simulink model "DC_Model_Collect"  (R2018a)
settings: Solver=VariableStepAuto  StartTime=0.0  StopTime=10.0  RelTol=1e-3
values from neighbouring files (symbols this model uses):
  A = [0 1 ; 0 -1]    [Ch8_18.m]    (also in Ch8_24.m = [-2 1; 0 -2]; Ch8_26.m = [1 0 ; 1 1]; DCT_3_3.m = find(abs(Zd)<0.05); DC_Model.m = [0 1 0; 0 -(B/J) Kt/J; 0 -(Ke/L) -(R/L)])
  a = 1:0.1:1.5    [Ch7_19.m]    (also in Ch7_25.m = (1-sin(th))/(1+sin(th)); DC_Model.m = 1)
  B = [1 ; 1]    [Ch8_18.m]    (also in Ch8_24.m = [1; 1]; Ch8_26.m = B0+expm(-A)*B1; DC_Model.m = 6.2e-05; NpointFFT.m = zeros(1,z-length(x)))
  B1 = [0; B]    [Ch8_24.m]    (also in Ch8_26.m = [0 ; 1]; DC_Model.m = [0; 0; 1/L])
  C = [2 1]    [Ch8_18.m]    (also in Ch8_24.m = [1 1]; Ch8_26.m = [1 1]; DC_Model.m = [1 0 0])
  J = 31*10^(-6)    (= 3.1e-05)    [DC_Model.m]
  Ka = 1/(3*Kp)    (= 0.0265223848928)    [DC_Model.m]
  Kas = 1/Kps    (= 110.951304705)    [DC_Model.m]
  Ke = 0.54    [DC_Model.m]
  Ki = R*1571    (= 3142)    [DC_Model.m]
  Kis = J*157^2/(5*Kt)    (= 0.283007037037)    [DC_Model.m]
  Kp = L*1571    (= 12.568)    [DC_Model.m]
  Kps = J*157/Kt    (= 0.00901296296296)    [DC_Model.m]
  Kps_1 = (1-a)*Kps    (= 0)    [DC_Model.m]
  Kt = 0.54    [DC_Model.m]
  L = 0.008    [DC_Model.m]
  posKa = 0    [DC_Model.m]
  posKd = 1    [DC_Model.m]
  posKi = 0    [DC_Model.m]
  posKp = 30    [DC_Model.m]
  R = 2    [Ch8_18.m]    (also in Ch8_26.m = 1; DC_Model.m)
undefined symbols (not defined in the file or in its folder): K
settings Model: Creator=admin  LastModifiedBy=admin

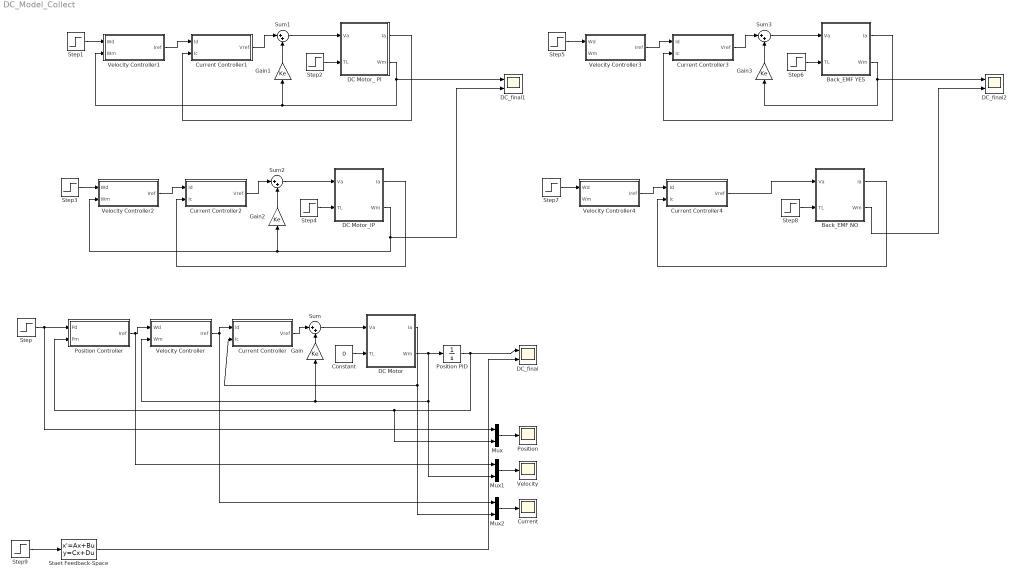
== system DC_Model_Collect ==
  Back_EMF NO : Subsystem
  Back_EMF YES : Subsystem
  Constant : Constant  Value=0
  Current : Scope
  Current Controller : Subsystem
  Current Controller1 : Subsystem
  Current Controller2 : Subsystem
  Current Controller3 : Subsystem
  Current Controller4 : Subsystem
  DC Motor : Subsystem
  DC Motor_ PI : Subsystem
  DC Motor_IP : Subsystem
  DC_final : Scope  NumInputPorts=2
  DC_final1 : Scope  NumInputPorts=2
  DC_final2 : Scope  NumInputPorts=2
  Gain{,1..3} (4 alike) : Gain  Gain=Ke
  Mux : Mux  Inputs=2
  Mux1 : Mux  Inputs=2
  Mux2 : Mux  Inputs=2
  Position : Scope
  Position Controller : Subsystem
  Position PID : Integrator
  Staet Feedback-Space : StateSpace  A=A-B1*K  B=B1  C=C  D=0  InitialCondition=0
  Step{,1,3,5,7,9} (6 alike) : Step  After=31.4  SampleTime=0
  Step{2,4,6,8} (4 alike) : Step  Time=2  After=0.1  SampleTime=0
  Sum{,1..3} (4 alike) : Sum  Inputs=|++
  Velocity : Scope
  Velocity Controller : Subsystem
  Velocity Controller1 : Subsystem
  Velocity Controller2 : Subsystem
  Velocity Controller3 : Subsystem
  Velocity Controller4 : Subsystem
  wires:
  Velocity Controller/1(Iref) -> Mux2/1, Current Controller/1(Id)
  DC Motor/2(Wm) -> Gain/1, Velocity Controller/2(Wm), Mux1/2, Position PID/1
  Position Controller/1(Iref) -> Mux1/1, Velocity Controller/1(Wd)
  Step/1 -> Mux/1, Position Controller/1(Pd)
  Position PID/1 -> DC_final/1, Position Controller/2(Pm), Mux/2
  DC Motor/1(Ia) -> Current Controller/2(Ic), Mux2/2
  Mux/1 -> Position/1
  Mux1/1 -> Velocity/1
  Mux2/1 -> Current/1
  Sum/1 -> DC Motor/1(Va)
  Gain/1 -> Sum/2
  Current Controller/1(Vref) -> Sum/1
  Sum1/1 -> DC Motor_ PI/1(Va)
  Step1/1 -> Velocity Controller1/1(Wd)
  Velocity Controller1/1(Iref) -> Current Controller1/1(Id)
  Current Controller1/1(Vref) -> Sum1/1
  Gain1/1 -> Sum1/2
  Step2/1 -> DC Motor_ PI/2(TL)
  DC Motor_ PI/1(Ia) -> Current Controller1/2(Ic)
  DC Motor_ PI/2(Wm) -> DC_final1/1, Gain1/1, Velocity Controller1/2(Wm)
  DC Motor_IP/2(Wm) -> DC_final1/2, Velocity Controller2/2(Wm), Gain2/1
  DC Motor_IP/1(Ia) -> Current Controller2/2(Ic)
  Step4/1 -> DC Motor_IP/2(TL)
  Gain2/1 -> Sum2/2
  Current Controller2/1(Vref) -> Sum2/1
  Velocity Controller2/1(Iref) -> Current Controller2/1(Id)
  Step3/1 -> Velocity Controller2/1(Wd)
  Sum2/1 -> DC Motor_IP/1(Va)
  Step7/1 -> Velocity Controller4/1(Wd)
  Velocity Controller4/1(Iref) -> Current Controller4/1(Id)
  Step8/1 -> Back_EMF NO/2(TL)
  Back_EMF NO/1(Ia) -> Current Controller4/2(Ic)
  Back_EMF NO/2(Wm) -> DC_final2/2
  Back_EMF YES/2(Wm) -> Gain3/1, DC_final2/1
  Back_EMF YES/1(Ia) -> Current Controller3/2(Ic)
  Step6/1 -> Back_EMF YES/2(TL)
  Gain3/1 -> Sum3/2
  Current Controller3/1(Vref) -> Sum3/1
  Velocity Controller3/1(Iref) -> Current Controller3/1(Id)
  Step5/1 -> Velocity Controller3/1(Wd)
  Sum3/1 -> Back_EMF YES/1(Va)
  Current Controller4/1(Vref) -> Back_EMF NO/1(Va)
  Step9/1 -> Staet Feedback-Space/1
  Constant/1 -> DC Motor/2(TL)
  Staet Feedback-Space/1 -> DC_final/2

== system DC_Model_Collect/Back_EMF NO ==
  Va : Inport
  TL : Inport  Port=2
  Gain : Gain  Gain=Kt
  Gain1 : Gain  Gain=Ke
  Sum : Sum  Inputs=|+-
  Sum1 : Sum  Inputs=-+|
  Transfer Fcn : TransferFcn  Denominator=[L R]
  Transfer Fcn1 : TransferFcn  Denominator=[J B]
  Ia : Outport
  Wm : Outport  Port=2
  wires:
  Va/1 -> Sum/1
  Transfer Fcn1/1 -> Wm/1, Gain1/1
  Sum/1 -> Transfer Fcn/1
  Gain/1 -> Sum1/2
  Sum1/1 -> Transfer Fcn1/1
  Gain1/1 -> Sum/2
  Transfer Fcn/1 -> Gain/1, Ia/1
  TL/1 -> Sum1/1

== system DC_Model_Collect/Back_EMF YES ==
  Va : Inport
  TL : Inport  Port=2
  Gain : Gain  Gain=Kt
  Gain1 : Gain  Gain=Ke
  Sum : Sum  Inputs=|+-
  Sum1 : Sum  Inputs=-+|
  Transfer Fcn : TransferFcn  Denominator=[L R]
  Transfer Fcn1 : TransferFcn  Denominator=[J B]
  Ia : Outport
  Wm : Outport  Port=2
  wires:
  TL/1 -> Sum1/1
  Transfer Fcn/1 -> Ia/1, Gain/1
  Gain1/1 -> Sum/2
  Sum1/1 -> Transfer Fcn1/1
  Gain/1 -> Sum1/2
  Sum/1 -> Transfer Fcn/1
  Transfer Fcn1/1 -> Gain1/1, Wm/1
  Va/1 -> Sum/1

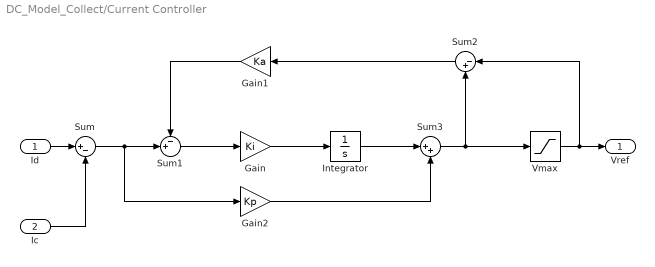
== system DC_Model_Collect/Current Controller ==
  Id : Inport
  Ic : Inport  Port=2
  Gain : Gain  Gain=Ki
  Gain1 : Gain  Gain=Ka
  Gain2 : Gain  Gain=Kp
  Integrator : Integrator
  Sum : Sum  Inputs=|+-
  Sum1 : Sum  Inputs=-+|
  Sum2 : Sum  Inputs=|-+
  Sum3 : Sum  Inputs=|++
  Vmax : Saturate  UpperLimit=200
  Vref : Outport
  wires:
  Id/1 -> Sum/1
  Sum1/1 -> Gain/1
  Ic/1 -> Sum/2
  Sum/1 -> Gain2/1, Sum1/2
  Gain1/1 -> Sum1/1
  Sum2/1 -> Gain1/1
  Vmax/1 -> Sum2/1, Vref/1
  Sum3/1 -> Sum2/2, Vmax/1
  Integrator/1 -> Sum3/1
  Gain/1 -> Integrator/1
  Gain2/1 -> Sum3/2

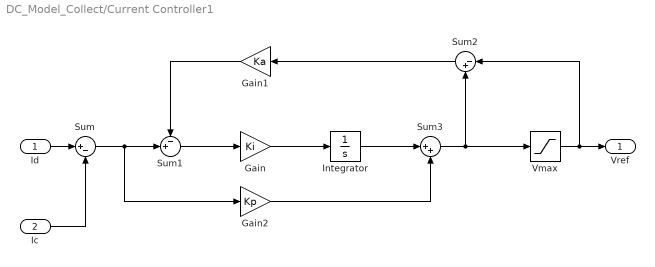
== system DC_Model_Collect/Current Controller1 ==
  Id : Inport
  Ic : Inport  Port=2
  Gain : Gain  Gain=Ki
  Gain1 : Gain  Gain=Ka
  Gain2 : Gain  Gain=Kp
  Integrator : Integrator
  Sum : Sum  Inputs=|+-
  Sum1 : Sum  Inputs=-+|
  Sum2 : Sum  Inputs=|-+
  Sum3 : Sum  Inputs=|++
  Vmax : Saturate  UpperLimit=300  LowerLimit=0
  Vref : Outport
  wires:
  Gain2/1 -> Sum3/2
  Gain/1 -> Integrator/1
  Integrator/1 -> Sum3/1
  Sum3/1 -> Vmax/1, Sum2/2
  Vmax/1 -> Vref/1, Sum2/1
  Sum2/1 -> Gain1/1
  Gain1/1 -> Sum1/1
  Sum/1 -> Sum1/2, Gain2/1
  Ic/1 -> Sum/2
  Sum1/1 -> Gain/1
  Id/1 -> Sum/1

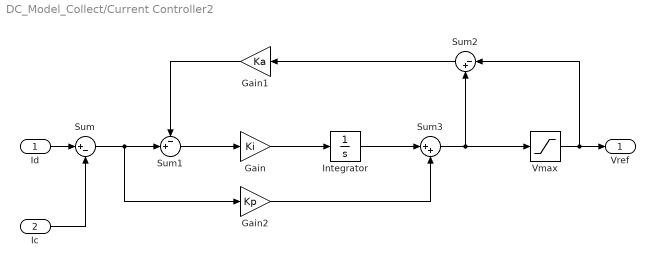
== system DC_Model_Collect/Current Controller2 ==
  Id : Inport
  Ic : Inport  Port=2
  Gain : Gain  Gain=Ki
  Gain1 : Gain  Gain=Ka
  Gain2 : Gain  Gain=Kp
  Integrator : Integrator
  Sum : Sum  Inputs=|+-
  Sum1 : Sum  Inputs=-+|
  Sum2 : Sum  Inputs=|-+
  Sum3 : Sum  Inputs=|++
  Vmax : Saturate  UpperLimit=300
  Vref : Outport
  wires:
  Id/1 -> Sum/1
  Sum1/1 -> Gain/1
  Ic/1 -> Sum/2
  Sum/1 -> Gain2/1, Sum1/2
  Gain1/1 -> Sum1/1
  Sum2/1 -> Gain1/1
  Vmax/1 -> Sum2/1, Vref/1
  Sum3/1 -> Sum2/2, Vmax/1
  Integrator/1 -> Sum3/1
  Gain/1 -> Integrator/1
  Gain2/1 -> Sum3/2

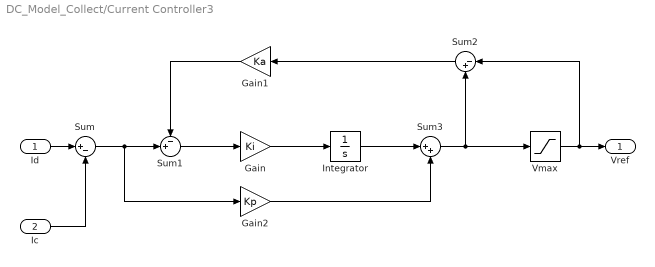
== system DC_Model_Collect/Current Controller3 ==
  Id : Inport
  Ic : Inport  Port=2
  Gain : Gain  Gain=Ki
  Gain1 : Gain  Gain=Ka
  Gain2 : Gain  Gain=Kp
  Integrator : Integrator
  Sum : Sum  Inputs=|+-
  Sum1 : Sum  Inputs=-+|
  Sum2 : Sum  Inputs=|-+
  Sum3 : Sum  Inputs=|++
  Vmax : Saturate  UpperLimit=300  LowerLimit=0
  Vref : Outport
  wires:
  Id/1 -> Sum/1
  Sum1/1 -> Gain/1
  Ic/1 -> Sum/2
  Sum/1 -> Gain2/1, Sum1/2
  Gain1/1 -> Sum1/1
  Sum2/1 -> Gain1/1
  Vmax/1 -> Sum2/1, Vref/1
  Sum3/1 -> Sum2/2, Vmax/1
  Integrator/1 -> Sum3/1
  Gain/1 -> Integrator/1
  Gain2/1 -> Sum3/2

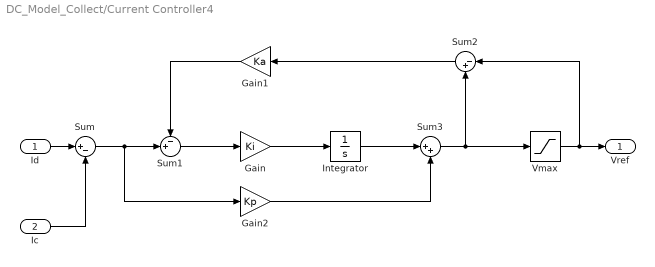
== system DC_Model_Collect/Current Controller4 ==
  Id : Inport
  Ic : Inport  Port=2
  Gain : Gain  Gain=Ki
  Gain1 : Gain  Gain=Ka
  Gain2 : Gain  Gain=Kp
  Integrator : Integrator
  Sum : Sum  Inputs=|+-
  Sum1 : Sum  Inputs=-+|
  Sum2 : Sum  Inputs=|-+
  Sum3 : Sum  Inputs=|++
  Vmax : Saturate  UpperLimit=300
  Vref : Outport
  wires:
  Gain2/1 -> Sum3/2
  Gain/1 -> Integrator/1
  Integrator/1 -> Sum3/1
  Sum3/1 -> Vmax/1, Sum2/2
  Vmax/1 -> Vref/1, Sum2/1
  Sum2/1 -> Gain1/1
  Gain1/1 -> Sum1/1
  Sum/1 -> Sum1/2, Gain2/1
  Ic/1 -> Sum/2
  Sum1/1 -> Gain/1
  Id/1 -> Sum/1

== system DC_Model_Collect/DC Motor ==
  Va : Inport
  TL : Inport  Port=2
  Gain : Gain  Gain=Kt
  Gain1 : Gain  Gain=Ke
  Sum : Sum  Inputs=|+-
  Sum1 : Sum  Inputs=-+|
  Transfer Fcn : TransferFcn  Denominator=[L R]
  Transfer Fcn1 : TransferFcn  Denominator=[J B]
  Ia : Outport
  Wm : Outport  Port=2
  wires:
  TL/1 -> Sum1/1
  Transfer Fcn/1 -> Ia/1, Gain/1
  Gain1/1 -> Sum/2
  Sum1/1 -> Transfer Fcn1/1
  Gain/1 -> Sum1/2
  Sum/1 -> Transfer Fcn/1
  Transfer Fcn1/1 -> Gain1/1, Wm/1
  Va/1 -> Sum/1

== system DC_Model_Collect/DC Motor_ PI ==
  Va : Inport
  TL : Inport  Port=2
  Gain : Gain  Gain=Kt
  Gain1 : Gain  Gain=Ke
  Sum : Sum  Inputs=|+-
  Sum1 : Sum  Inputs=-+|
  Transfer Fcn : TransferFcn  Denominator=[L R]
  Transfer Fcn1 : TransferFcn  Denominator=[J B]
  Ia : Outport
  Wm : Outport  Port=2
  wires:
  Va/1 -> Sum/1
  Transfer Fcn1/1 -> Wm/1, Gain1/1
  Sum/1 -> Transfer Fcn/1
  Gain/1 -> Sum1/2
  Sum1/1 -> Transfer Fcn1/1
  Gain1/1 -> Sum/2
  Transfer Fcn/1 -> Gain/1, Ia/1
  TL/1 -> Sum1/1

== system DC_Model_Collect/DC Motor_IP ==
  Va : Inport
  TL : Inport  Port=2
  Gain : Gain  Gain=Kt
  Gain1 : Gain  Gain=Ke
  Sum : Sum  Inputs=|+-
  Sum1 : Sum  Inputs=-+|
  Transfer Fcn : TransferFcn  Denominator=[L R]
  Transfer Fcn1 : TransferFcn  Denominator=[J B]
  Ia : Outport
  Wm : Outport  Port=2
  wires:
  TL/1 -> Sum1/1
  Transfer Fcn/1 -> Ia/1, Gain/1
  Gain1/1 -> Sum/2
  Sum1/1 -> Transfer Fcn1/1
  Gain/1 -> Sum1/2
  Sum/1 -> Transfer Fcn/1
  Transfer Fcn1/1 -> Gain1/1, Wm/1
  Va/1 -> Sum/1

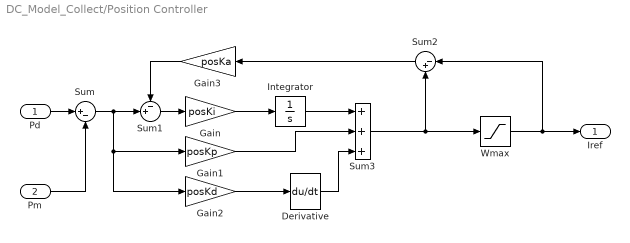
== system DC_Model_Collect/Position Controller ==
  Pd : Inport
  Pm : Inport  Port=2
  Derivative : Derivative
  Gain : Gain  Gain=posKi
  Gain1 : Gain  Gain=posKp
  Gain2 : Gain  Gain=posKd
  Gain3 : Gain  Gain=posKa
  Integrator : Integrator
  Sum : Sum  Inputs=|+-
  Sum1 : Sum  Inputs=-+|
  Sum2 : Sum  Inputs=|-+
  Sum3 : Sum  Inputs=+++
  Wmax : Saturate  UpperLimit=100  LowerLimit=-100
  Iref : Outport
  wires:
  Pm/1 -> Sum/2
  Pd/1 -> Sum/1
  Sum/1 -> Gain2/1, Gain1/1, Sum1/2
  Sum1/1 -> Gain/1
  Gain/1 -> Integrator/1
  Gain2/1 -> Derivative/1
  Wmax/1 -> Sum2/1, Iref/1
  Sum2/1 -> Gain3/1
  Gain3/1 -> Sum1/1
  Integrator/1 -> Sum3/1
  Gain1/1 -> Sum3/2
  Derivative/1 -> Sum3/3
  Sum3/1 -> Sum2/2, Wmax/1

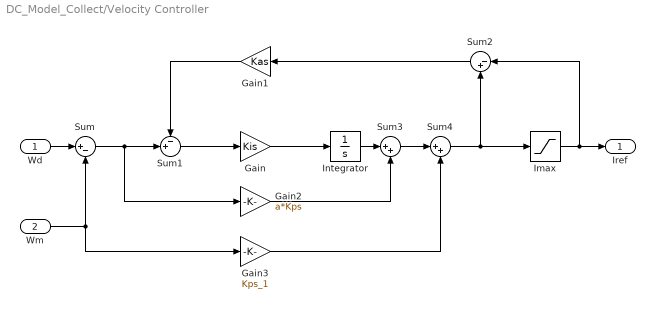
== system DC_Model_Collect/Velocity Controller ==
  Wd : Inport
  Wm : Inport  Port=2
  Gain : Gain  Gain=Kis
  Gain1 : Gain  Gain=Kas
  Gain2 : Gain  Gain=a*Kps
  Gain3 : Gain  Gain=Kps_1
  Imax : Saturate  UpperLimit=20
  Integrator : Integrator
  Sum : Sum  Inputs=|+-
  Sum1 : Sum  Inputs=-+|
  Sum2 : Sum  Inputs=|-+
  Sum3 : Sum  Inputs=|++
  Sum4 : Sum  Inputs=|++
  Iref : Outport
  wires:
  Gain2/1 -> Sum3/2
  Gain/1 -> Integrator/1
  Integrator/1 -> Sum3/1
  Imax/1 -> Iref/1, Sum2/1
  Sum2/1 -> Gain1/1
  Gain1/1 -> Sum1/1
  Sum/1 -> Sum1/2, Gain2/1
  Sum1/1 -> Gain/1
  Wd/1 -> Sum/1
  Wm/1 -> Gain3/1, Sum/2
  Gain3/1 -> Sum4/2
  Sum3/1 -> Sum4/1
  Sum4/1 -> Sum2/2, Imax/1

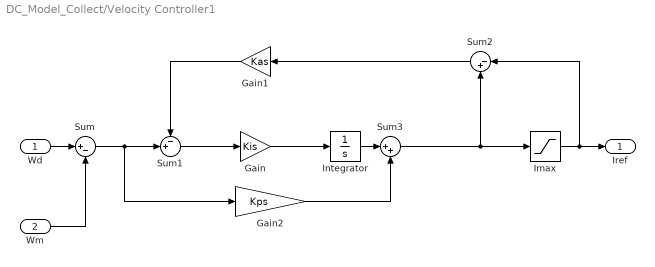
== system DC_Model_Collect/Velocity Controller1 ==
  Wd : Inport
  Wm : Inport  Port=2
  Gain : Gain  Gain=Kis
  Gain1 : Gain  Gain=Kas
  Gain2 : Gain  Gain=Kps
  Imax : Saturate  UpperLimit=20  LowerLimit=0
  Integrator : Integrator
  Sum : Sum  Inputs=|+-
  Sum1 : Sum  Inputs=-+|
  Sum2 : Sum  Inputs=|-+
  Sum3 : Sum  Inputs=|++
  Iref : Outport
  wires:
  Sum3/1 -> Imax/1, Sum2/2
  Wm/1 -> Sum/2
  Wd/1 -> Sum/1
  Sum1/1 -> Gain/1
  Sum/1 -> Gain2/1, Sum1/2
  Gain1/1 -> Sum1/1
  Sum2/1 -> Gain1/1
  Imax/1 -> Sum2/1, Iref/1
  Integrator/1 -> Sum3/1
  Gain/1 -> Integrator/1
  Gain2/1 -> Sum3/2

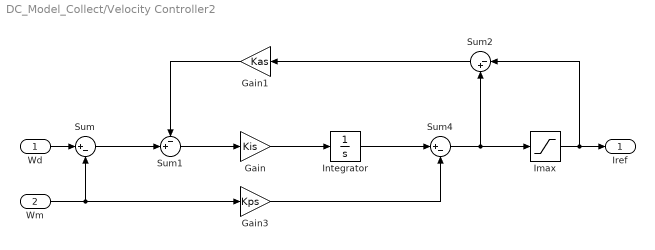
== system DC_Model_Collect/Velocity Controller2 ==
  Wd : Inport
  Wm : Inport  Port=2
  Gain : Gain  Gain=Kis
  Gain1 : Gain  Gain=Kas
  Gain3 : Gain  Gain=Kps
  Imax : Saturate  UpperLimit=20  LowerLimit=-20
  Integrator : Integrator
  Sum : Sum  Inputs=|+-
  Sum1 : Sum  Inputs=-+|
  Sum2 : Sum  Inputs=|-+
  Sum4 : Sum  Inputs=|+-
  Iref : Outport
  wires:
  Gain/1 -> Integrator/1
  Integrator/1 -> Sum4/1
  Imax/1 -> Iref/1, Sum2/1
  Sum2/1 -> Gain1/1
  Gain1/1 -> Sum1/1
  Sum/1 -> Sum1/2
  Sum1/1 -> Gain/1
  Wd/1 -> Sum/1
  Wm/1 -> Gain3/1, Sum/2
  Gain3/1 -> Sum4/2
  Sum4/1 -> Sum2/2, Imax/1

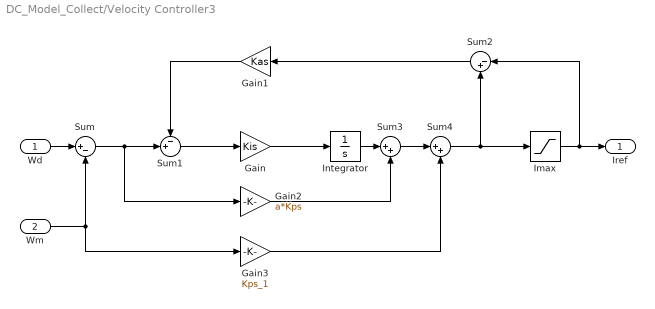
== system DC_Model_Collect/Velocity Controller3 ==
  Wd : Inport
  Wm : Inport  Port=2
  Gain : Gain  Gain=Kis
  Gain1 : Gain  Gain=Kas
  Gain2 : Gain  Gain=a*Kps
  Gain3 : Gain  Gain=Kps_1
  Imax : Saturate  UpperLimit=20  LowerLimit=0
  Integrator : Integrator
  Sum : Sum  Inputs=|+-
  Sum1 : Sum  Inputs=-+|
  Sum2 : Sum  Inputs=|-+
  Sum3 : Sum  Inputs=|++
  Sum4 : Sum  Inputs=|++
  Iref : Outport
  wires:
  Gain2/1 -> Sum3/2
  Gain/1 -> Integrator/1
  Integrator/1 -> Sum3/1
  Imax/1 -> Iref/1, Sum2/1
  Sum2/1 -> Gain1/1
  Gain1/1 -> Sum1/1
  Sum/1 -> Sum1/2, Gain2/1
  Sum1/1 -> Gain/1
  Wd/1 -> Sum/1
  Wm/1 -> Gain3/1, Sum/2
  Gain3/1 -> Sum4/2
  Sum3/1 -> Sum4/1
  Sum4/1 -> Sum2/2, Imax/1

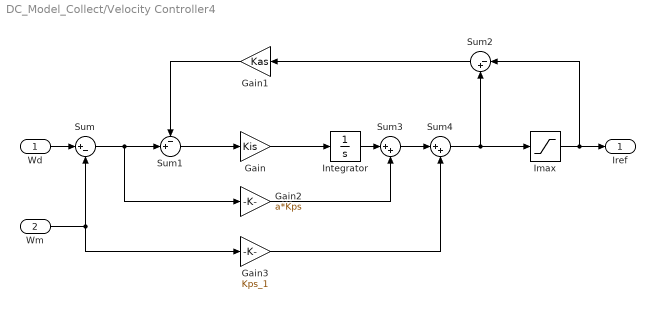
== system DC_Model_Collect/Velocity Controller4 ==
  Wd : Inport
  Wm : Inport  Port=2
  Gain : Gain  Gain=Kis
  Gain1 : Gain  Gain=Kas
  Gain2 : Gain  Gain=a*Kps
  Gain3 : Gain  Gain=Kps_1
  Imax : Saturate  UpperLimit=20  LowerLimit=0
  Integrator : Integrator
  Sum : Sum  Inputs=|+-
  Sum1 : Sum  Inputs=-+|
  Sum2 : Sum  Inputs=|-+
  Sum3 : Sum  Inputs=|++
  Sum4 : Sum  Inputs=|++
  Iref : Outport
  wires:
  Sum4/1 -> Imax/1, Sum2/2
  Sum3/1 -> Sum4/1
  Gain3/1 -> Sum4/2
  Wm/1 -> Sum/2, Gain3/1
  Wd/1 -> Sum/1
  Sum1/1 -> Gain/1
  Sum/1 -> Gain2/1, Sum1/2
  Gain1/1 -> Sum1/1
  Sum2/1 -> Gain1/1
  Imax/1 -> Sum2/1, Iref/1
  Integrator/1 -> Sum3/1
  Gain/1 -> Integrator/1
  Gain2/1 -> Sum3/2
